simulink model "Process"  (R2023a)
settings: Solver=FixedStepDiscrete  StartTime=0.0  StopTime=0.  FixedStep=1.0  RelTol=1e-3
settings Model: Creator=horty  LastModifiedBy=horty
settings DataIOCC: SaveFormat=Array  SignalLogging=off  DSMLogging=off  SaveTime=off  ReturnWorkspaceOutputs=off

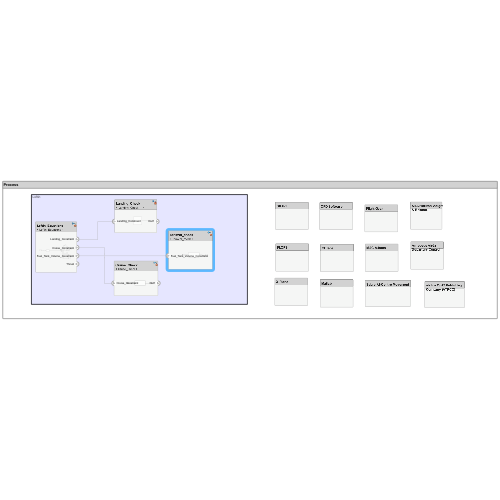
[thumbnail: Simulink's stored preview of the top-level diagram]
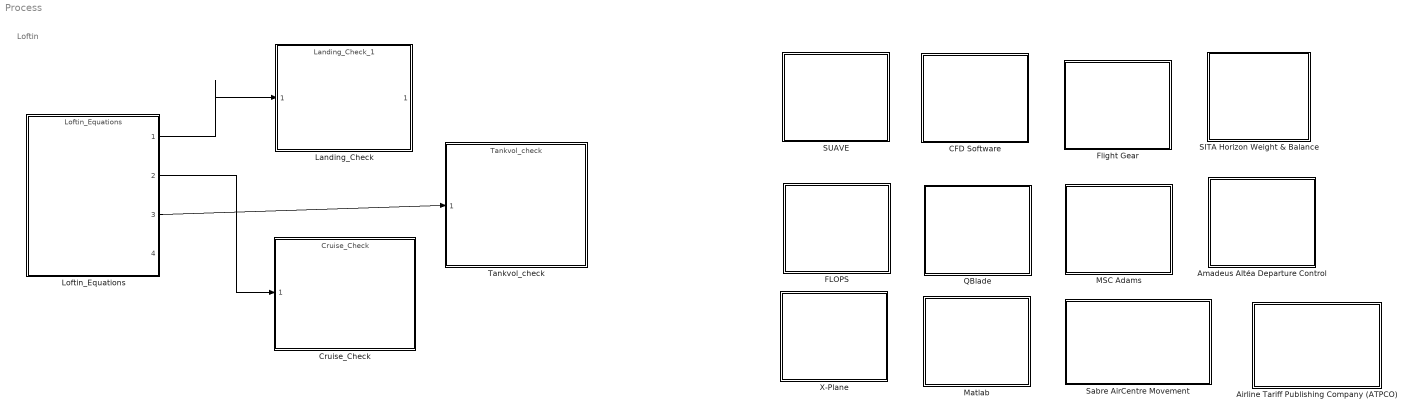
== system Process ==
  note: Loftin
  Airline Tariff Publishing Company (ATPCO) : Subsystem
      settings: PortSchema="{\"entries\":[{\"content\":{\"headerSize\":26,\"margin\":15,\"minimumSpacing\":25,\"sides\":[{\"content\":{},\"type\":\"ConnectorPlacement.EquallySpacedRectSide\",\"uuid\":\"636d2f87-93d9-45fd-9aeb-9aaf83ba7ed3\"},{\"content\":{\"side\":\"RIGHT\"},\"type\":\"ConnectorPlacement.EquallySpacedRectSide\",\"uuid\":\"cf2237c5-0aa6-4654-9855-d204880971d0\"},{\"content\":{\"side\":\"TOP\"},\"type\":\"ConnectorPlacement.EquallySpacedRectSide\",\"uuid\":\"9c6cf233-afb4-45ef-a06e-ee533b0b1896\"}]},\"type\":\"ConnectorPlacement.EquallySpacedConnector\",\"uuid\":\"b836bcaf-28f0-4381-b4b6-d91ee18d608f\"}],\"packageUris\":[\"http://schema.mathworks.com/mf0/Connector/R2020b\"],\"version\":\"1.0\"}"
  Amadeus Altéa Departure Control : Subsystem
      settings: PortSchema="{\"entries\":[{\"content\":{\"headerSize\":26,\"margin\":15,\"minimumSpacing\":25,\"sides\":[{\"content\":{},\"type\":\"ConnectorPlacement.EquallySpacedRectSide\",\"uuid\":\"636d2f87-93d9-45fd-9aeb-9aaf83ba7ed3\"},{\"content\":{\"side\":\"RIGHT\"},\"type\":\"ConnectorPlacement.EquallySpacedRectSide\",\"uuid\":\"cf2237c5-0aa6-4654-9855-d204880971d0\"},{\"content\":{\"side\":\"TOP\"},\"type\":\"ConnectorPlacement.EquallySpacedRectSide\",\"uuid\":\"9c6cf233-afb4-45ef-a06e-ee533b0b1896\"}]},\"type\":\"ConnectorPlacement.EquallySpacedConnector\",\"uuid\":\"b836bcaf-28f0-4381-b4b6-d91ee18d608f\"}],\"packageUris\":[\"http://schema.mathworks.com/mf0/Connector/R2020b\"],\"version\":\"1.0\"}"
  CFD Software : Subsystem
      settings: PortSchema="{\"entries\":[{\"content\":{\"headerSize\":26,\"margin\":15,\"minimumSpacing\":25,\"sides\":[{\"content\":{},\"type\":\"ConnectorPlacement.EquallySpacedRectSide\",\"uuid\":\"636d2f87-93d9-45fd-9aeb-9aaf83ba7ed3\"},{\"content\":{\"side\":\"RIGHT\"},\"type\":\"ConnectorPlacement.EquallySpacedRectSide\",\"uuid\":\"cf2237c5-0aa6-4654-9855-d204880971d0\"},{\"content\":{\"side\":\"TOP\"},\"type\":\"ConnectorPlacement.EquallySpacedRectSide\",\"uuid\":\"9c6cf233-afb4-45ef-a06e-ee533b0b1896\"}]},\"type\":\"ConnectorPlacement.EquallySpacedConnector\",\"uuid\":\"b836bcaf-28f0-4381-b4b6-d91ee18d608f\"}],\"packageUris\":[\"http://schema.mathworks.com/mf0/Connector/R2020b\"],\"version\":\"1.0\"}"
  Cruise_Check : ModelReference  ModelNameDialog=Cruise_Check  SimulationMode=Normal  ModelReferenceVersion=1.6
      settings: PortSchema="{\"entries\":[{\"content\":{\"headerSize\":38,\"margin\":15,\"minimumSpacing\":25,\"sides\":[{\"content\":{\"connectorIds\":[\"In1\"]},\"type\":\"ConnectorPlacement.EquallySpacedRectSide\",\"uuid\":\"622bfa65-fc3f-4eab-b03f-2882386ec589\"},{\"content\":{\"side\":\"RIGHT\"},\"type\":\"ConnectorPlacement.EquallySpacedRectSide\",\"uuid\":\"e967c2b2-b23d-4224-b744-09ef492c395e\"},{\"content\":{\"side\":\"TOP\"},\"type\":\"ConnectorPlacement.EquallySpacedRectSide\",\"uuid\":\"d03612cc-6593-4126-abaf-60b42808215f\"}]},\"type\":\"ConnectorPlacement.EquallySpacedConnector\",\"uuid\":\"874feb9c-09b6-46d0-94b5-09f3ffac4bac\"}],\"packageUris\":[\"http://schema.mathworks.com/mf0/Connector/R2020b\"],\"version\":\"1.0\"}"
  FLOPS : Subsystem
      settings: PortSchema="{\"entries\":[{\"content\":{\"headerSize\":26,\"margin\":15,\"minimumSpacing\":25,\"sides\":[{\"content\":{},\"type\":\"ConnectorPlacement.EquallySpacedRectSide\",\"uuid\":\"4e80462b-46b4-4a98-8f84-5df78bae93bd\"},{\"content\":{\"side\":\"RIGHT\"},\"type\":\"ConnectorPlacement.EquallySpacedRectSide\",\"uuid\":\"1cf8eeff-6f52-4041-ac5a-fe93b20bd07d\"},{\"content\":{\"side\":\"TOP\"},\"type\":\"ConnectorPlacement.EquallySpacedRectSide\",\"uuid\":\"f4111f56-95eb-408d-b258-f048dea1611d\"}]},\"type\":\"ConnectorPlacement.EquallySpacedConnector\",\"uuid\":\"d404d3e1-bef5-4a3c-ab17-8392e1c270c9\"}],\"packageUris\":[\"http://schema.mathworks.com/mf0/Connector/R2020b\"],\"version\":\"1.0\"}"
  Flight Gear : Subsystem
      settings: PortSchema="{\"entries\":[{\"content\":{\"headerSize\":26,\"margin\":15,\"minimumSpacing\":25,\"sides\":[{\"content\":{},\"type\":\"ConnectorPlacement.EquallySpacedRectSide\",\"uuid\":\"636d2f87-93d9-45fd-9aeb-9aaf83ba7ed3\"},{\"content\":{\"side\":\"RIGHT\"},\"type\":\"ConnectorPlacement.EquallySpacedRectSide\",\"uuid\":\"cf2237c5-0aa6-4654-9855-d204880971d0\"},{\"content\":{\"side\":\"TOP\"},\"type\":\"ConnectorPlacement.EquallySpacedRectSide\",\"uuid\":\"9c6cf233-afb4-45ef-a06e-ee533b0b1896\"}]},\"type\":\"ConnectorPlacement.EquallySpacedConnector\",\"uuid\":\"b836bcaf-28f0-4381-b4b6-d91ee18d608f\"}],\"packageUris\":[\"http://schema.mathworks.com/mf0/Connector/R2020b\"],\"version\":\"1.0\"}"
  Landing_Check : ModelReference  ModelNameDialog=Landing_Check_1  SimulationMode=Normal  ModelReferenceVersion=1.7
      settings: PortSchema="{\"entries\":[{\"content\":{\"headerSize\":38,\"margin\":15,\"minimumSpacing\":25,\"sides\":[{\"content\":{\"connectorIds\":[\"In1\"]},\"type\":\"ConnectorPlacement.EquallySpacedRectSide\",\"uuid\":\"622bfa65-fc3f-4eab-b03f-2882386ec589\"},{\"content\":{\"connectorIds\":[\"Out1\"],\"side\":\"RIGHT\"},\"type\":\"ConnectorPlacement.EquallySpacedRectSide\",\"uuid\":\"e967c2b2-b23d-4224-b744-09ef492c395e\"},{\"content\":{\"side\":\"TOP\"},\"type\":\"ConnectorPlacement.EquallySpacedRectSide\",\"uuid\":\"d03612cc-6593-4126-abaf-60b42808215f\"}]},\"type\":\"ConnectorPlacement.EquallySpacedConnector\",\"uuid\":\"874feb9c-09b6-46d0-94b5-09f3ffac4bac\"}],\"packageUris\":[\"http://schema.mathworks.com/mf0/Connector/R2020b\"],\"version\":\"1.0\"}"
  Loftin_Equations : ModelReference  ModelNameDialog=Loftin_Equations  SimulationMode=Normal  ModelReferenceVersion=1.9
      settings: PortSchema="{\"entries\":[{\"content\":{\"headerSize\":38,\"margin\":15,\"minimumSpacing\":25,\"sides\":[{\"content\":{},\"type\":\"ConnectorPlacement.EquallySpacedRectSide\",\"uuid\":\"4e80462b-46b4-4a98-8f84-5df78bae93bd\"},{\"content\":{\"connectorIds\":[\"Out1\",\"Out2\",\"Out3\",\"Out4\"],\"side\":\"RIGHT\"},\"type\":\"ConnectorPlacement.EquallySpacedRectSide\",\"uuid\":\"1cf8eeff-6f52-4041-ac5a-fe93b20bd07d\"},{\"content\":{\"side\":\"TOP\"},\"type\":\"ConnectorPlacement.EquallySpacedRectSide\",\"uuid\":\"f4111f56-95eb-408d-b258-f048dea1611d\"}]},\"type\":\"ConnectorPlacement.EquallySpacedConnector\",\"uuid\":\"d404d3e1-bef5-4a3c-ab17-8392e1c270c9\"}],\"packageUris\":[\"http://schema.mathworks.com/mf0/Connector/R2020b\"],\"version\":\"1.0\"}"
  MSC Adams : Subsystem
      settings: PortSchema="{\"entries\":[{\"content\":{\"headerSize\":26,\"margin\":15,\"minimumSpacing\":25,\"sides\":[{\"content\":{},\"type\":\"ConnectorPlacement.EquallySpacedRectSide\",\"uuid\":\"636d2f87-93d9-45fd-9aeb-9aaf83ba7ed3\"},{\"content\":{\"side\":\"RIGHT\"},\"type\":\"ConnectorPlacement.EquallySpacedRectSide\",\"uuid\":\"cf2237c5-0aa6-4654-9855-d204880971d0\"},{\"content\":{\"side\":\"TOP\"},\"type\":\"ConnectorPlacement.EquallySpacedRectSide\",\"uuid\":\"9c6cf233-afb4-45ef-a06e-ee533b0b1896\"}]},\"type\":\"ConnectorPlacement.EquallySpacedConnector\",\"uuid\":\"b836bcaf-28f0-4381-b4b6-d91ee18d608f\"}],\"packageUris\":[\"http://schema.mathworks.com/mf0/Connector/R2020b\"],\"version\":\"1.0\"}"
  Matlab : Subsystem
      settings: PortSchema="{\"entries\":[{\"content\":{\"headerSize\":26,\"margin\":15,\"minimumSpacing\":25,\"sides\":[{\"content\":{},\"type\":\"ConnectorPlacement.EquallySpacedRectSide\",\"uuid\":\"636d2f87-93d9-45fd-9aeb-9aaf83ba7ed3\"},{\"content\":{\"side\":\"RIGHT\"},\"type\":\"ConnectorPlacement.EquallySpacedRectSide\",\"uuid\":\"cf2237c5-0aa6-4654-9855-d204880971d0\"},{\"content\":{\"side\":\"TOP\"},\"type\":\"ConnectorPlacement.EquallySpacedRectSide\",\"uuid\":\"9c6cf233-afb4-45ef-a06e-ee533b0b1896\"}]},\"type\":\"ConnectorPlacement.EquallySpacedConnector\",\"uuid\":\"b836bcaf-28f0-4381-b4b6-d91ee18d608f\"}],\"packageUris\":[\"http://schema.mathworks.com/mf0/Connector/R2020b\"],\"version\":\"1.0\"}"
  QBlade : Subsystem
      settings: PortSchema="{\"entries\":[{\"content\":{\"headerSize\":26,\"margin\":15,\"minimumSpacing\":25,\"sides\":[{\"content\":{},\"type\":\"ConnectorPlacement.EquallySpacedRectSide\",\"uuid\":\"636d2f87-93d9-45fd-9aeb-9aaf83ba7ed3\"},{\"content\":{\"side\":\"RIGHT\"},\"type\":\"ConnectorPlacement.EquallySpacedRectSide\",\"uuid\":\"cf2237c5-0aa6-4654-9855-d204880971d0\"},{\"content\":{\"side\":\"TOP\"},\"type\":\"ConnectorPlacement.EquallySpacedRectSide\",\"uuid\":\"9c6cf233-afb4-45ef-a06e-ee533b0b1896\"}]},\"type\":\"ConnectorPlacement.EquallySpacedConnector\",\"uuid\":\"b836bcaf-28f0-4381-b4b6-d91ee18d608f\"}],\"packageUris\":[\"http://schema.mathworks.com/mf0/Connector/R2020b\"],\"version\":\"1.0\"}"
  SITA Horizon Weight & Balance : Subsystem
      settings: PortSchema="{\"entries\":[{\"content\":{\"headerSize\":26,\"margin\":15,\"minimumSpacing\":25,\"sides\":[{\"content\":{},\"type\":\"ConnectorPlacement.EquallySpacedRectSide\",\"uuid\":\"636d2f87-93d9-45fd-9aeb-9aaf83ba7ed3\"},{\"content\":{\"side\":\"RIGHT\"},\"type\":\"ConnectorPlacement.EquallySpacedRectSide\",\"uuid\":\"cf2237c5-0aa6-4654-9855-d204880971d0\"},{\"content\":{\"side\":\"TOP\"},\"type\":\"ConnectorPlacement.EquallySpacedRectSide\",\"uuid\":\"9c6cf233-afb4-45ef-a06e-ee533b0b1896\"}]},\"type\":\"ConnectorPlacement.EquallySpacedConnector\",\"uuid\":\"b836bcaf-28f0-4381-b4b6-d91ee18d608f\"}],\"packageUris\":[\"http://schema.mathworks.com/mf0/Connector/R2020b\"],\"version\":\"1.0\"}"
  SUAVE : Subsystem
      settings: PortSchema="{\"entries\":[{\"content\":{\"headerSize\":26,\"margin\":15,\"minimumSpacing\":25,\"sides\":[{\"content\":{},\"type\":\"ConnectorPlacement.EquallySpacedRectSide\",\"uuid\":\"4e80462b-46b4-4a98-8f84-5df78bae93bd\"},{\"content\":{\"side\":\"RIGHT\"},\"type\":\"ConnectorPlacement.EquallySpacedRectSide\",\"uuid\":\"1cf8eeff-6f52-4041-ac5a-fe93b20bd07d\"},{\"content\":{\"side\":\"TOP\"},\"type\":\"ConnectorPlacement.EquallySpacedRectSide\",\"uuid\":\"f4111f56-95eb-408d-b258-f048dea1611d\"}]},\"type\":\"ConnectorPlacement.EquallySpacedConnector\",\"uuid\":\"d404d3e1-bef5-4a3c-ab17-8392e1c270c9\"}],\"packageUris\":[\"http://schema.mathworks.com/mf0/Connector/R2020b\"],\"version\":\"1.0\"}"
  Sabre AirCentre Movement : Subsystem
      settings: PortSchema="{\"entries\":[{\"content\":{\"headerSize\":26,\"margin\":15,\"minimumSpacing\":25,\"sides\":[{\"content\":{},\"type\":\"ConnectorPlacement.EquallySpacedRectSide\",\"uuid\":\"636d2f87-93d9-45fd-9aeb-9aaf83ba7ed3\"},{\"content\":{\"side\":\"RIGHT\"},\"type\":\"ConnectorPlacement.EquallySpacedRectSide\",\"uuid\":\"cf2237c5-0aa6-4654-9855-d204880971d0\"},{\"content\":{\"side\":\"TOP\"},\"type\":\"ConnectorPlacement.EquallySpacedRectSide\",\"uuid\":\"9c6cf233-afb4-45ef-a06e-ee533b0b1896\"}]},\"type\":\"ConnectorPlacement.EquallySpacedConnector\",\"uuid\":\"b836bcaf-28f0-4381-b4b6-d91ee18d608f\"}],\"packageUris\":[\"http://schema.mathworks.com/mf0/Connector/R2020b\"],\"version\":\"1.0\"}"
  Tankvol_check : ModelReference  ModelNameDialog=Tankvol_check  SimulationMode=Normal  ModelReferenceVersion=1.8
      settings: PortSchema="{\"entries\":[{\"content\":{\"headerSize\":38,\"margin\":15,\"minimumSpacing\":25,\"sides\":[{\"content\":{\"connectorIds\":[\"In1\"]},\"type\":\"ConnectorPlacement.EquallySpacedRectSide\",\"uuid\":\"622bfa65-fc3f-4eab-b03f-2882386ec589\"},{\"content\":{\"side\":\"RIGHT\"},\"type\":\"ConnectorPlacement.EquallySpacedRectSide\",\"uuid\":\"e967c2b2-b23d-4224-b744-09ef492c395e\"},{\"content\":{\"side\":\"TOP\"},\"type\":\"ConnectorPlacement.EquallySpacedRectSide\",\"uuid\":\"d03612cc-6593-4126-abaf-60b42808215f\"}]},\"type\":\"ConnectorPlacement.EquallySpacedConnector\",\"uuid\":\"874feb9c-09b6-46d0-94b5-09f3ffac4bac\"}],\"packageUris\":[\"http://schema.mathworks.com/mf0/Connector/R2020b\"],\"version\":\"1.0\"}"
  X-Plane : Subsystem
      settings: PortSchema="{\"entries\":[{\"content\":{\"headerSize\":26,\"margin\":15,\"minimumSpacing\":25,\"sides\":[{\"content\":{},\"type\":\"ConnectorPlacement.EquallySpacedRectSide\",\"uuid\":\"636d2f87-93d9-45fd-9aeb-9aaf83ba7ed3\"},{\"content\":{\"side\":\"RIGHT\"},\"type\":\"ConnectorPlacement.EquallySpacedRectSide\",\"uuid\":\"cf2237c5-0aa6-4654-9855-d204880971d0\"},{\"content\":{\"side\":\"TOP\"},\"type\":\"ConnectorPlacement.EquallySpacedRectSide\",\"uuid\":\"9c6cf233-afb4-45ef-a06e-ee533b0b1896\"}]},\"type\":\"ConnectorPlacement.EquallySpacedConnector\",\"uuid\":\"b836bcaf-28f0-4381-b4b6-d91ee18d608f\"}],\"packageUris\":[\"http://schema.mathworks.com/mf0/Connector/R2020b\"],\"version\":\"1.0\"}"
  wires:
  Loftin_Equations/1 -> Landing_Check/1
  Loftin_Equations/2 -> Cruise_Check/1
  Loftin_Equations/3 -> Tankvol_check/1

== system Process/Airline Tariff Publishing Company (ATPCO) ==

== system Process/Amadeus Altéa Departure Control ==

== system Process/CFD Software ==

== system Process/FLOPS ==

== system Process/Flight Gear ==

== system Process/MSC Adams ==

== system Process/Matlab ==

== system Process/QBlade ==

== system Process/SITA Horizon Weight & Balance ==

== system Process/SUAVE ==

== system Process/Sabre AirCentre Movement ==

== system Process/X-Plane ==
